simulink model "OBCSystem"  (R2025b)
settings: Solver=FixedStepAuto  StartTime=0.0  StopTime=100e-3  RelTol=1e-3  EnableMultiTasking=on
PreLoadFcn:
  | %% Load OBCSystem initialization parameters
  | initScriptPath = fullfile(fileparts(which('OBCSystem')), '..', 'SupportFiles', 'Scripts', 'OBCSystem_init.m');
  | if isfile(initScriptPath)
  |     evalin('base', fileread(initScriptPath));
  | else
  |     warning('OBCSystem:initNotFound', 'OBCSystem_init.m not found at: %s', initScriptPath);
  | end
InitFcn:
  | mode = str2double(get_param('OBCSystem/System/SimulationMode','value'));
  | enableLogging = str2double(get_param('OBCSystem/System/On-Board Charger/HIL/EnableHighResLogging','value'));
  | 
  | % If the charger runs on the FPGA AND high-resolution logging is enabled,
  | % uncomment interrupt setup. Comment otherwise
  | if ((mode == 2) && (enableLogging == 1))
  |     set_param('OBCSystem/Interrupt Setup','Commented','off');
  | else
  |     set_param('OBCSystem/Interrupt Setup','Commented','on');
  | end
  | 
  | % If DMA streaming is enambled and simulation time exceeds 30s, then throw an error
  | maxStopTime = 30;   % seconds
  | stopTimeStr = get_param(bdroot, 'StopTime');
  | stopTimeVal = str2double(stopTimeStr);
  | 
  | if enableLogging && stopTimeVal > maxStopTime
  |     error('DMA streaming is enabled, but StopTime = %.3f s exceeds the allowed %.3f s.', ...
  |           stopTimeVal, maxStopTime);
  | end
undefined symbols (not defined in the file): DAB, DAB_CCCV_Ki, DAB_CCCV_Kp, DAB_CCCV_Kt, DAB_Charging, DAB_CurrentReference, DAB_DCOffset, DAB_PhaseShift_LowerSat, DAB_PhaseShift_UpperSat, DAB_PhaseShiftInit, DAB_PhaseToDeg, DAB_PID_Kd, DAB_PID_Ki, DAB_PID_Kp, DAB_PID_LowerSat, DAB_PID_N, DAB_PID_UpperSat, Fourier_class, FPGA, FrameSize, getfullname, grid, Instr_EffGain, Instr_PinGain, Instr_PoutGain, Instr_pUtoDeg, Instr_RippleGain, Instr_SoCGain, IO334, Ki_current, Ki_voltage, Kp_current, Kp_voltage, MIL_or_HIL, OBC_template1, OpenLoopDuty, OpenLoopEnable, PCIe_RT, PFC_Current_Kb, PFC_Current_LowerSat, PFC_Current_UpperSat, PFC_Sat_DC_Lower, PFC_Sat_DC_Upper, PFC_Sat_iL_Lower, PFC_Sat_iL_Upper, PFC_Sat_Pwr_Lower, PFC_Sat_Pwr_Upper, PFC_Voltage_Kb, PFC_Voltage_LowerSat, PFC_Voltage_UpperSat, Rblock, Real, Time, totemPole, ts_CPU, ts_FPGA_clk, ts_FPGA_mdl, VectorSize
libraries: nesl_utility x27, fl_lib x24, speedgoatlib_hdlCoder_IO3xx x20, ee_lib x12, simulink x4, eeGeneralControl x4, slpidlib x3, pwm_cpulib x2, batteryecm_lib x2, slrealtimeloglib x2, pwm_fpgalib x2, speedgoatlib_interrupt x1
(part 1 of 4)
settings Model: ExtModeEnableFloating=off  ExtModeTrigDuration=100000  Creator=The MathWorks, Inc.  LastModifiedBy=aldiyar.semedyarov
settings SolverCC: ConcurrentTasks=on  AlgebraicLoopSolver=TrustRegion  PositivePriorityOrder=on  InsertRTBMode=Never (minimum delay)
settings DataIOCC: SaveFormat=Array  SaveState=on  LoggingFileName=OBCSystem_log
settings OptimizationCC: BlockReduction=off  BooleanDataType=off  GainParamInheritBuiltInType=on  OptimizeBlockIOStorage=off  BufferReuse=off  ReuseModelBlockBuffer=off  GlobalBufferReuse=off  ExpressionFolding=off  LocalBlockOutputs=off  InitFltsAndDblsToZero=on  OptimizeDataStoreBuffers=off  BusAssignmentInplaceUpdate=off
settings DebuggingCC: SaveWithParameterizedLinksMsg=none  UnderspecifiedInitializationDetection=Classic  MergeDetectMultiDrivingBlocksExec=none  CheckExecutionContextPreStartOutputMsg=on  SignalResolutionControl=TryResolveAllWithWarning  InheritedTsInSrcMsg=none  TasksWithSamePriorityMsg=none  UnconnectedInputMsg=warning  UnconnectedOutputMsg=warning  UnconnectedLineMsg=warning  SFUnexpectedBacktrackingDiag=warning  SFNoUnconditionalDefaultTransitionDiag=warning  SFExecutionAtInitializationDiag=none  ArithmeticOperatorsInVariantConditions=warning
settings HardwareCC: ProdBitPerLong=64.0  ProdLongLongMode=on  ProdHWDeviceType=Intel->x86-64 (Linux 64)
settings ModelReferenceCC: EnableRefExpFcnMdlSchedulingChecks=on  PropagateSignalLabelsOutOfModel=off
settings SFSimCC: SimUseLocalCustomCode=off  CustomCodeUndefinedFunction=UseInterfaceOnly
settings RTWCC: SystemTargetFile=speedgoat.tlc  TemplateMakefile=slrealtime_default_tmf  RTWUseLocalCustomCode=off  Toolchain=Simulink Real-Time Toolchain  BuildConfiguration=Faster Runs  CodeExecutionProfiling=on  TargetLang=C++  GPUComputeCapability=3.5  Description=Speedgoat Real-Time Target Machine
settings CodeAppCC: StateflowObjectComments=on
settings SimulinkRealTimeTargetCC: SLRTFileLogMaxRuns=1.0  ExtModeMaxTrigDuration=10.0  ExtModeStaticAllocSize=1000000.0  ExtModeTransport=0.0  MultiwordLength=2048.0  DynamicStringBufferSize=256.0  PreserveMATLABNamespacesInGeneratedCode=on  SubcomponentCodeInterfacePackaging=Reusable function  MATLABClassNameForMDSCustomization=Simulink.SoftwareTarget.GRTCustomization  InstructionSetFMA=off  LogToMDFFile=off
settings ConfigComp: CovMetricSettings=dw  CovSaveCumulativeToWorkspaceVar=on  CovSaveSingleToWorkspaceVar=on  CovExternalEMLEnable=off  CovSFcnEnable=off

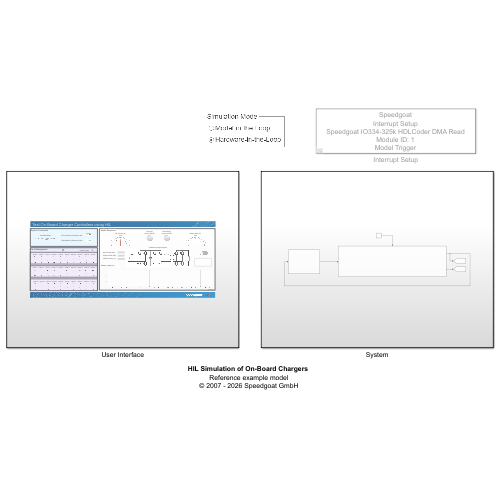
[thumbnail: Simulink's stored preview of the top-level diagram]
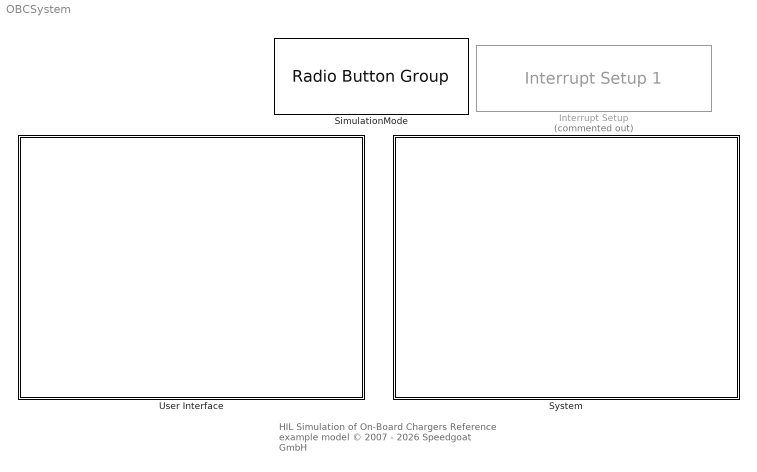
== system OBCSystem ==
  note: HIL Simulation of On-Board Chargers
      | Reference example model
      | © 2007 - 2026 Speedgoat GmbH
  Interrupt Setup : speedgoatlib_interrupt/Interrupt Setup 1  Commented=on  parModuleTrigger=on  parPollingMode=off  parPriorityConf=High  parPriority=253  confStartFcn=IO334_325K_HDLC_DMA_READ_start_public  confStopFcn=IO334_325K_HDLC_DMA_READ_stop_public  confIsrFcn=IO334_325K_HDLC_DMA_READ_isr_public  confMapFcn=IO334_325K_HDLC_DMA_READ_map_public  confHookFile=io334_325k_hdlc_dma_read_int_hooks.c  confIrqNr=-1  confIsPolling=off  confModID=16776961  confSelectedInt=Speedgoat IO334-325k HDLCoder DMA Read  confSelectedId=1  confSelectedChannel=[]  confData=[90 1]  confForcePollingMode=off
  SimulationMode : RadioButtonGroup  LabelPosition=Hide  SelectedLabel=Hardware-in-the-Loop  ButtonGroupName=Simulation Mode
  System : Subsystem
  User Interface : Subsystem

== system OBCSystem/System ==
  Controller : Subsystem
  On-Board Charger : Subsystem  Variant=on  VariantControl=Choice
      settings: PortSchema="{\"entries\":[{\"content\":{\"sides\":[{\"content\":{\"connectorIds\":[\"In1\"]},\"type\":\"ConnectorPlacement.EquallySpacedRectSide\",\"uuid\":\"470e74a6-3489-4910-833e-9935ca68db72\"},{\"content\":{\"connectorIds\":[\"Out1\",\"Out2\"],\"side\":\"RIGHT\"},\"type\":\"ConnectorPlacement.EquallySpacedRectSide\",\"uuid\":\"2bffa5e5-f1a3-4939-a790-ed9d5415056f\"},{\"content\":{\"connectorIds\":[\"In2\"],\"side\":\"TOP\"},\"type\":\"ConnectorPlacement.EquallySpacedRectSide\",\"uuid\":\"16820d5e-786f-42c5-b0ca-13ece32c30be\"}]},\"type\":\"ConnectorPlacement.EquallySpacedConnector\",\"uuid\":\"b4a77eb5-3b93-4396-97dc-6ff44775ea65\"}],\"packageUris\":[\"http://schema.mathworks.com/mf0/Connector/R2020b\"],\"version\":\"1.0\"}"
      mask Display: image('OnboardChargerSchematics.png');
  SimulationMode : Constant  Value=2  OutDataTypeStr=single  SampleTime=ts_CPU
  tag scope: Meas_bus2=global, Meas_bus=global
  wires:
  Controller/1(PWM_bus) -> On-Board Charger/1(PWM_bus)
  SimulationMode/1 -> On-Board Charger/2(Mode)
  On-Board Charger/1(Meas_bus) -> [Meas_bus], Controller/1(Meas_bus)
  On-Board Charger/2(Meas_bus2) -> [Meas_bus2]

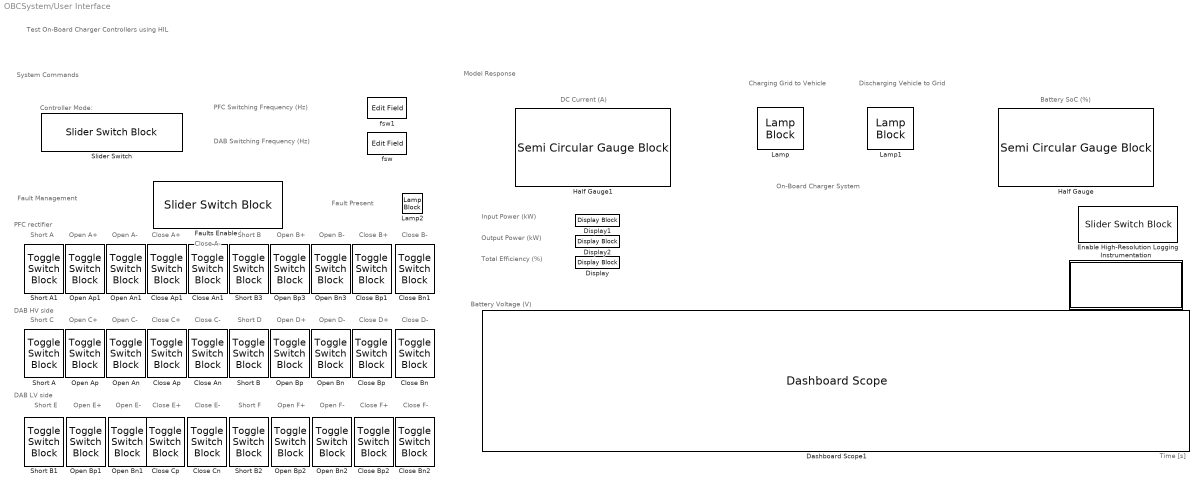
== system OBCSystem/User Interface ==
  note: Open C-
  note: PFC rectifier
  note: Open E-
  note: System Commands
  note: Short E
  note: Close D+
  note: Short F
  note: Discharging
      | Vehicle to Grid
  note: Model Response
  note: Close E-
  note: DC Current (A)
  note: Fault Present
  note: Charging
      | Grid to Vehicle
  note: Controller Mode:
  note: DAB HV side
  note: Open F-
  note: Battery Voltage (V)
  note: Open D-
  note: On-Board Charger System
  note: Open E+
  note: Close C+
  note: Close D-
  note: Fault Management
  note: DAB Switching Frequency (Hz)
  note: Short C
  note: Short D
  note: Close A-
  note: Battery SoC (%)
  note: Open B+
  note: Short A
  note: Close A+
  note: Close B+
  note: Short B
  note: Time [s]
  note: Close F-
  note: DAB LV side
  note: Open F+
  note: Open D+
  note: Close C-
  note: Open B-
  note: Close B-
  note: Close E+
  note: Open A+
  note: Open A-
  note: Close F+
  note: Test On-Board Charger Controllers using HIL
  note: PFC Switching Frequency (Hz)
  note: Open C+
  note: Total Efficiency (%)
  note: Input Power (kW)
  note: Output Power (kW)
  Close An : ToggleSwitchBlock  LabelPosition=Hide
  Close An1 : ToggleSwitchBlock  LabelPosition=Hide
  Close Ap : ToggleSwitchBlock  LabelPosition=Hide
  Close Ap1 : ToggleSwitchBlock  LabelPosition=Hide
  Close Bn : ToggleSwitchBlock  LabelPosition=Hide
  Close Bn1 : ToggleSwitchBlock  LabelPosition=Hide
  Close Bn2 : ToggleSwitchBlock  LabelPosition=Hide
  Close Bp : ToggleSwitchBlock  LabelPosition=Hide
  Close Bp1 : ToggleSwitchBlock  LabelPosition=Hide
  Close Bp2 : ToggleSwitchBlock  LabelPosition=Hide
  Close Cn : ToggleSwitchBlock  LabelPosition=Hide
  Close Cp : ToggleSwitchBlock  LabelPosition=Hide
  Dashboard Scope1 : DashboardScope  ShowInitialText=off  TimeSpan=45  Ymin=385  Ymax=402.5  ScaleAtStop=off  FontColor=[0.0, 0.0, 0.0]
  Display : DisplayBlock  LabelPosition=Hide  Transparency=1  GridColor=[0.502, 0.502, 0.502]
  Display1 : DisplayBlock  LabelPosition=Hide  Transparency=1  GridColor=[0.502, 0.502, 0.502]
  Display2 : DisplayBlock  LabelPosition=Hide  Transparency=1  GridColor=[0.502, 0.502, 0.502]
  Enable High-Resolution Logging : SliderSwitchBlock  LabelPosition=Hide
  Faults Enabled : SliderSwitchBlock  LabelPosition=Hide
  Half Gauge : SemiCircularGaugeBlock  LabelPosition=Hide  FontColor=[0.0, 0.0, 0.0]
  Half Gauge1 : SemiCircularGaugeBlock  LabelPosition=Hide  ScaleMin=-20  ScaleMax=20  FontColor=[0.0, 0.0, 0.0]
  Instrumentation : Subsystem
  Lamp : LampBlock  LabelPosition=Hide  DefaultColor=[192.0, 192.0, 192.0]
  Lamp1 : LampBlock  LabelPosition=Hide  DefaultColor=[192.0, 192.0, 192.0]
  Lamp2 : LampBlock  LabelPosition=Hide  DefaultColor=[192.0, 192.0, 192.0]
  Open An : ToggleSwitchBlock  LabelPosition=Hide
  Open An1 : ToggleSwitchBlock  LabelPosition=Hide
  Open Ap : ToggleSwitchBlock  LabelPosition=Hide
  Open Ap1 : ToggleSwitchBlock  LabelPosition=Hide
  Open Bn{,1..3} (4 alike) : ToggleSwitchBlock  LabelPosition=Hide
  Open Bp{,1..3} (4 alike) : ToggleSwitchBlock  LabelPosition=Hide
  Short A : ToggleSwitchBlock  LabelPosition=Hide
  Short A1 : ToggleSwitchBlock  LabelPosition=Hide
  Short B{,1..3} (4 alike) : ToggleSwitchBlock  LabelPosition=Hide
  Slider Switch : SliderSwitchBlock  LabelPosition=Hide
  fsw : EditField  LabelPosition=Hide  ShowInitialText=on  Alignment=Center
  fsw1 : EditField  LabelPosition=Hide  ShowInitialText=on  Alignment=Center

== system OBCSystem/System/Controller ==
  Meas_bus : Inport
  Bus Creator : BusCreator  Inputs=4
  Bus Selector : BusSelector  OutputSignals=VCbus,iL_PFC,Vs,Ibatt,Vbatt
  DAB Controller : Subsystem
  Ibatt_ref : Constant  Value=DAB_CurrentReference  OutDataTypeStr=double  SampleTime=ts_CPU
  PFC Controller : Subsystem
  PFC Reference DC Voltage : Constant  Value=400  OutDataTypeStr=single  SampleTime=ts_CPU
  PWM_bus : Outport
  tag scope: Ibatt_ref=global, Vdc_ref=global
  wires:
  Bus Selector/2 -> PFC Controller/3(Measured inductor current)  "<iL_PFC>"
  PFC Reference DC Voltage/1 -> [Vdc_ref]
  Bus Selector/3 -> PFC Controller/4(Source voltage)  "<Vs>"
  Bus Selector/5 -> DAB Controller/2(Measured battery voltage)  "<Vbatt>"
  Meas_bus/1 -> Bus Selector/1
  Bus Selector/1 -> PFC Controller/2(Measured bus voltage)  "<VCbus>"
  [Vdc_ref] -> PFC Controller/1(Reference bus voltage)
  PFC Controller/1(PWM_Config_PFC) -> Bus Creator/1  "PWM_Config_PFC"
  PFC Controller/2(PWM_Runtime_PFC) -> Bus Creator/2  "PWM_Runtime_PFC"
  DAB Controller/1(PWM_Config_DAB) -> Bus Creator/3  "PWM_Config_DAB"
  DAB Controller/2(PWM_Runtime_DAB) -> Bus Creator/4  "PWM_Runtime_DAB"
  Bus Creator/1 -> PWM_bus/1
  Ibatt_ref/1 -> [Ibatt_ref]
  [Ibatt_ref] -> DAB Controller/3(Reference battery current)
  Bus Selector/4 -> DAB Controller/1(Measured battery current)  "<Ibatt>"

== system OBCSystem/System/On-Board Charger ==
  PWM_bus : Inport
  Mode : Inport  Port=2
  HIL : Subsystem  VariantControl=strcmp(get_param('OBCSystem/System/SimulationMode','value'),'2')
  MIL : Subsystem  VariantControl=strcmp(get_param('OBCSystem/System/SimulationMode','value'),'1')
  Meas_bus : Outport
  Meas_bus2 : Outport  Port=2

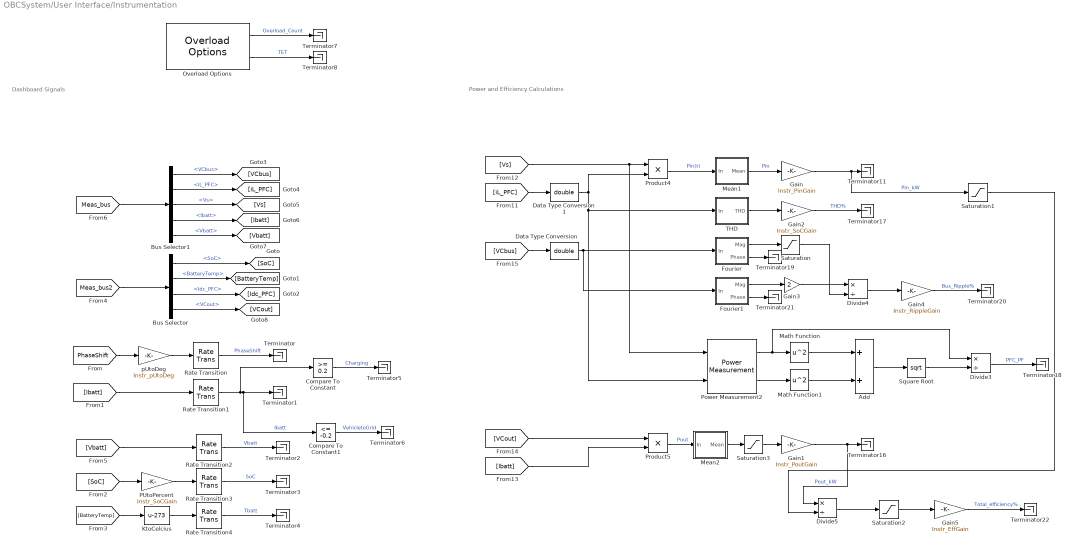
== system OBCSystem/User Interface/Instrumentation ==
  note: Dashboard Signals
  note: Power and Efficiency Calculations
  Add : Sum
  Bus Selector : BusSelector  OutputSignals=SoC,BatteryTemp,Idc_PFC,VCout
  Bus Selector1 : BusSelector  OutputSignals=VCbus,iL_PFC,Vs,Ibatt,Vbatt
  Compare To Constant : simulink/Logic and Bit Operations/Compare To Constant  relop=>=  const=0.2  OutDataTypeStr=boolean
  Compare To Constant1 : simulink/Logic and Bit Operations/Compare To Constant  relop=<=  const=-0.2  OutDataTypeStr=boolean
  Data Type Conversion : DataTypeConversion  OutDataTypeStr=double  SaturateOnIntegerOverflow=off  RndMeth=Floor
  Data Type Conversion1 : DataTypeConversion  OutDataTypeStr=double  SaturateOnIntegerOverflow=off  RndMeth=Floor
  Divide3 : Product  Inputs=*/
  Divide4 : Product  Inputs=*/
  Divide5 : Product  Inputs=*/
  Fourier : Subsystem
      settings: OpenFcn=elec.conv.unmask(gcb);
  Fourier1 : Subsystem
  Gain : Gain  Gain=Instr_PinGain
  Gain1 : Gain  Gain=Instr_PoutGain
  Gain2 : Gain  Gain=Instr_SoCGain
  Gain3 : Gain  Gain=2
  Gain4 : Gain  Gain=Instr_RippleGain
  Gain5 : Gain  Gain=Instr_EffGain
  KtoCelcius : Bias  Bias=-273  SaturateOnIntegerOverflow=off
  Math Function : Math  Operator=square
  Math Function1 : Math  Operator=square
  Mean1 : Subsystem
  Mean2 : Subsystem
      settings: OpenFcn=elec.conv.unmask(gcb);
  Overload Options : slrealtimetgmanagement/Overload Options  startupDur=1  startupDurSrc=Tunable Parameter  maxOverload=100  maxOverloadSrc=Tunable Parameter  TETFlag=on
  PUtoPercent : Gain  Gain=Instr_SoCGain
  Power Measurement2 : eePowerMeasurement/Power Measurement  LabelModeActiveChoice=Discrete  F=50  K=1  Ts=ts_CPU
  Product4 : Product  OutDataTypeStr=double
  Product5 : Product  OutDataTypeStr=double
  Rate Transition : RateTransition  OutPortSampleTime=1e-3
  Rate Transition1 : RateTransition  OutPortSampleTime=1e-3
  Rate Transition2 : RateTransition  InitialCondition=386  OutPortSampleTime=1e-3
  Rate Transition3 : RateTransition  InitialCondition=0.75  OutPortSampleTime=1e-3
  Rate Transition4 : RateTransition  InitialCondition=20  OutPortSampleTime=1e-3
  Saturation : Saturate  UpperLimit=inf  LowerLimit=eps
  Saturation1 : Saturate  UpperLimit=inf  LowerLimit=eps
  Saturation2 : Saturate  UpperLimit=1  LowerLimit=0
  Saturation3 : Saturate  UpperLimit=inf  LowerLimit=0
  Square Root : Sqrt
  THD : Subsystem
  Terminator{,1..8,11,16..22} (17 alike) : Terminator
  pUtoDeg : Gain  Gain=Instr_pUtoDeg
  wires:
  [PhaseShift] -> pUtoDeg/1
  [Ibatt] -> Rate Transition1/1
  [Vbatt] -> Rate Transition2/1
  Rate Transition/1 -> Terminator/1  "PhaseShift"
  Rate Transition1/1 -> Compare To Constant/1, Compare To Constant1/1, Terminator1/1  "Ibatt"
  Rate Transition2/1 -> Terminator2/1  "Vbatt"
  Rate Transition3/1 -> Terminator3/1  "SoC"
  pUtoDeg/1 -> Rate Transition/1
  [SoC] -> PUtoPercent/1
  [BatteryTemp] -> KtoCelcius/1
  Rate Transition4/1 -> Terminator4/1  "Tbatt"
  KtoCelcius/1 -> Rate Transition4/1
  Compare To Constant/1 -> Terminator5/1  "Charging"
  Compare To Constant1/1 -> Terminator6/1  "VehicletoGrid"
  PUtoPercent/1 -> Rate Transition3/1
  Overload Options/1 -> Terminator7/1  "Overload_Count"
  Overload Options/2 -> Terminator8/1  "TET"
  [Vs] -> Power Measurement2/1, Product4/1
  [iL_PFC] -> Data Type Conversion1/1
  Mean1/1(Mean) -> Gain/1  "Pin"
  Product4/1 -> Mean1/1(In)  "Pin(t)"
  Gain/1 -> Saturation1/1, Terminator11/1  "Pin_kW"
  Gain1/1 -> Divide5/1, Terminator16/1  "Pout_kW"
  [Ibatt] -> Product5/2
  [VCout] -> Product5/1
  THD/1(THD) -> Gain2/1
  Gain2/1 -> Terminator17/1  "THD%"
  Power Measurement2/1 -> Divide3/1, Math Function/1
  Math Function/1 -> Add/1
  Power Measurement2/2 -> Math Function1/1
  Math Function1/1 -> Add/2
  Add/1 -> Square Root/1
  Square Root/1 -> Divide3/2
  Divide3/1 -> Terminator18/1  "PFC_PF"
  [VCbus] -> Data Type Conversion/1
  Fourier/1(Mag) -> Saturation/1
  Fourier/2(Phase) -> Terminator19/1
  Gain3/1 -> Divide4/1
  Saturation/1 -> Divide4/2
  Fourier1/1(Mag) -> Gain3/1
  Divide4/1 -> Gain4/1
  Gain4/1 -> Terminator20/1  "Bus_Ripple%"
  Fourier1/2(Phase) -> Terminator21/1
  Data Type Conversion/1 -> Fourier1/1(In), Fourier/1(In)
  Data Type Conversion1/1 -> Power Measurement2/2, THD/1(In), Product4/2
  Divide5/1 -> Saturation2/1
  Gain5/1 -> Terminator22/1  "Total_efficiency%"
  Saturation2/1 -> Gain5/1
  Saturation1/1 -> Divide5/2
  [Meas_bus2] -> Bus Selector/1
  Bus Selector/1 -> [SoC]  "<SoC>"
  Bus Selector/2 -> [BatteryTemp]  "<BatteryTemp>"
  Bus Selector/3 -> [Idc_PFC]  "<Idc_PFC>"
  [Meas_bus] -> Bus Selector1/1
  Bus Selector1/1 -> [VCbus]  "<VCbus>"
  Bus Selector1/2 -> [iL_PFC]  "<iL_PFC>"
  Bus Selector1/3 -> [Vs]  "<Vs>"
  Bus Selector1/4 -> [Ibatt]  "<Ibatt>"
  Bus Selector1/5 -> [Vbatt]  "<Vbatt>"
  Bus Selector/4 -> [VCout]  "<VCout>"
  Product5/1 -> Mean2/1(In)  "Pout"
  Mean2/1(Mean) -> Saturation3/1
  Saturation3/1 -> Gain1/1

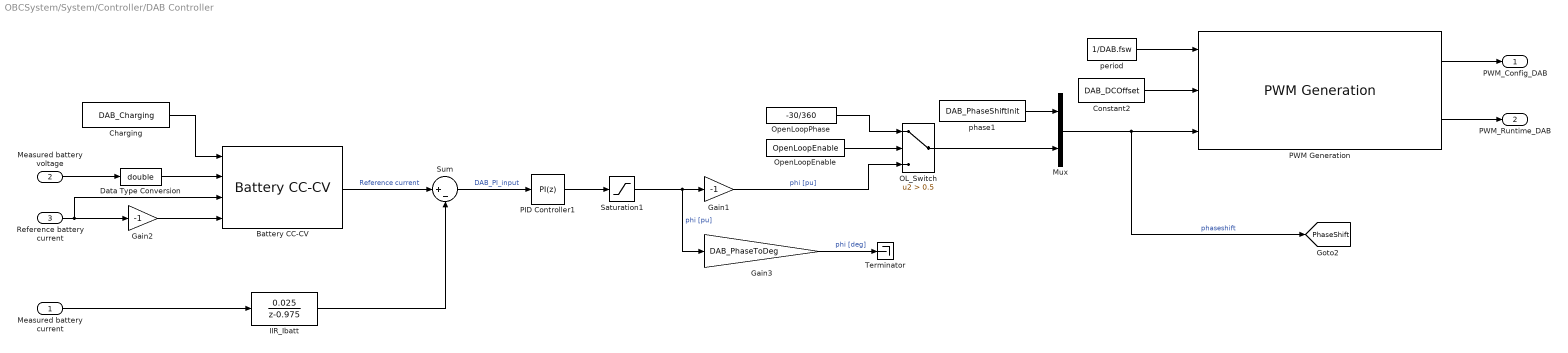
== system OBCSystem/System/Controller/DAB Controller ==
  Measured battery current : Inport
  Measured battery voltage : Inport  Port=2
  Reference battery current : Inport  Port=3
  Battery CC-CV : BatteryCurrentManagement/Battery CC-CV  MinMaxFlag=off  MaxCellVoltage=MaxCellVoltage  Kp=DAB_CCCV_Kp  Ki=DAB_CCCV_Ki  Kaw=DAB_CCCV_Kaw  Kt=DAB_CCCV_Kt  Ts=-1
      settings: LibrarySourceBlock=batt_sl_lib/Current Management/Battery CC-CV
  Charging : Constant  Value=DAB_Charging  SampleTime=ts_CPU
  Constant2 : Constant  Value=DAB_DCOffset  SampleTime=-1
  Data Type Conversion : DataTypeConversion  OutDataTypeStr=double  SaturateOnIntegerOverflow=off  RndMeth=Floor
  Gain1 : Gain  Gain=-1
  Gain2 : Gain  Gain=-1
  Gain3 : Gain  Gain=DAB_PhaseToDeg
  IIR_Ibatt : DiscreteTransferFcn  Numerator=[0.025]  Denominator=[1, -0.975]  SampleTime=ts_CPU
  Mux : Mux  Inputs=2
  OL_Switch : Switch  Criteria=u2 > Threshold  Threshold=0.5  SaturateOnIntegerOverflow=off  InputSameDT=off
  OpenLoopEnable : Constant  Value=OpenLoopEnable  SampleTime=ts_CPU
  OpenLoopPhase : Constant  Value=-30/360  SampleTime=ts_CPU
  PID Controller1 : slpidlib/PID Controller  Controller=PI  Form=Parallel  TimeDomain=Discrete-time  UseExternalTs=off  SampleTime=ts_CPU  IntegratorMethod=Forward Euler  FilterMethod=Forward Euler  ControllerParametersSource=internal  P=DAB_PID_Kp  I=DAB_PID_Ki  UseKiTs=off  D=DAB_PID_Kd  UseExternalDerivativeSource=off  N=DAB_PID_N  UseFilter=on  TunerSelectOption=Transfer Function Based (PID Tuner App)  InitialConditionSource=internal  InitialConditionForIntegrator=0  InitialConditionForFilter=0  DifferentiatorICPrevScaledInput=0  ExternalReset=none  TrackingMode=off  Kt=1  LimitOutput=on  SatLimitsSource=internal  UpperSaturationLimit=DAB_PID_UpperSat  LowerSaturationLimit=DAB_PID_LowerSat  LinearizeAsGain=on  AntiWindupMode=clamping  Kb=1  LimitIntegrator=off  UpperIntegratorSaturationLimit=inf  LowerIntegratorSaturationLimit=-inf  POutMin=[]  POutMax=[]  IOutMin=[]  IOutMax=[]  DOutMin=[]  DOutMax=[]  NOutMin=[]  NOutMax=[]  SumOutMin=[]  SumOutMax=[]  SaturationOutMin=[]  SaturationOutMax=[]  PParamMin=[]  PParamMax=[]  IParamMin=[]  IParamMax=[]  DParamMin=[]  DParamMax=[]  NParamMin=[]  NParamMax=[]  KbParamMin=[]  KbParamMax=[]  KtParamMin=[]  KtParamMax=[]  KbOutMin=[]  KbOutMax=[]  KtOutMin=[]  KtOutMax=[]  IntegratorOutMin=[]  IntegratorOutMax=[]  FilterOutMin=[]  FilterOutMax=[]  SumI1OutMin=[]  SumI1OutMax=[]  SumI2OutMin=[]  SumI2OutMax=[]  SumI3OutMin=[]  SumI3OutMax=[]  SumI4OutMin=[]  SumI4OutMax=[]  SumDOutMin=[]  SumDOutMax=[]  DifferentiatorOutMin=[]  DifferentiatorOutMax=[]  FilterDiffOutCoefMin=[]  FilterDiffOutCoefMax=[]  ReciprocalOutMin=[]  ReciprocalOutMax=[]  SumDenOutMin=[]  SumDenOutMax=[]  SumNumOutMin=[]  SumNumOutMax=[]  DivideOutMin=[]  DivideOutMax=[]  UdiffTsProdOutMin=[]  UdiffTsProdOutMax=[]  NTsProdOutMin=[]  NTsProdOutMax=[]  UintegralTsProdOutMin=[]  UintegralTsProdOutMax=[]  UngainTsProdOutMin=[]  UngainTsProdOutMax=[]  ClampingZeroOutDataTypeStr=Inherit: Inherit via back propagation  ClampingZeroOutMin=[]  ClampingZeroOutMax=[]  FilterDenConstantOutDataTypeStr=Inherit: Inherit via back propagation  FilterDenConstantOutMin=[]  FilterDenConstantOutMax=[]  PCopyOutDataTypeStr=Inherit: Inherit via back propagation  PCopyOutMin=[]  PCopyOutMax=[]  NCopyOutDataTypeStr=Inherit: Inherit via back propagation  NCopyOutMin=[]  NCopyOutMax=[]  IntegratorContinuousStateAttributes=''  IntegratorStateMustResolveToSignalObject=off  IntegratorRTWStateStorageClass=Auto  FilterContinuousStateAttributes=''  FilterStateMustResolveToSignalObject=off  FilterRTWStateStorageClass=Auto  ParallelPVariant=InternalParameters  IdealPVariant=Disabled  IVariant=InternalParameters  DVariant=Disabled  IntegratorVariant=Discrete  SatVariant=Enabled  AWVariant=DiscClampingParallel  PCopyVariant=Disabled  TRVariant=Disabled  FdbkBlocksVariant=Forward  IdealPFdbkVariant=Disabled  SatFdbkVariant=Disabled  DerivativeFilterVariant=Disabled  NVariant=Disabled  NCopyVariant=Disabled_SignalSpec  FilterICVariant=Disabled  IntegratorICVariant=InternalICs  ExternalResetVariant=Disabled  TRSumVariant=Passthrough  SumFdbkVariant=Disabled  SumVariant=Sum_PI  TsampFilterVariant=InternalTs  TsampNgainVariant=Passthrough  TsampIntegralVariant=Disabled_SignalSpec  ExternalSaturationOutDataTypeStr=Inherit: Same as second input  DerivativeSourceVariant=Disabled  PreIntVariant=InternalPreInt
  PWM Generation : pwm_cpulib/PWM Generation  f_FPGA=1/ts_FPGA_clk  n_channels=2  sel_scaling=CPU  protection_param=B is forced off when A is on.  deadband_sec=DAB_PWM_Deadband  natural_update=At period starts  delay=0  trigger_duration_sec=[1e-6]  trigger_period_start=off  trigger_half_of_the_period=off  trigger_a_on=off  trigger_a_off=off  trigger_b_on=off  trigger_b_off=off  bit_width_pwm_gen=DAB_PWM_BitWidth  invert_a=off  invert_b=off  invert_c=off  showPhaseInput=on
      settings: SourceProductName=PWM CPU Library
  Saturation1 : Saturate  UpperLimit=DAB_PhaseShift_UpperSat  LowerLimit=DAB_PhaseShift_LowerSat
  Sum : Sum  Inputs=|+-
  Terminator : Terminator
  period : Constant  Value=1/DAB.fsw  SampleTime=-1
  phase1 : Constant  Value=DAB_PhaseShiftInit  SampleTime=-1
  PWM_Config_DAB : Outport  VectorParamsAs1DForOutWhenUnconnected=off
  PWM_Runtime_DAB : Outport  Port=2  VectorParamsAs1DForOutWhenUnconnected=off
  tag scope: PhaseShift=global
  wires:
  Sum/1 -> PID Controller1/1  "DAB_PI_input"
  Saturation1/1 -> Gain1/1, Gain3/1  "phi [pu]"
  PID Controller1/1 -> Saturation1/1
  Measured battery current/1 -> IIR_Ibatt/1
  Gain3/1 -> Terminator/1  "phi [deg]"
  period/1 -> PWM Generation/1
  phase1/1 -> Mux/1
  Mux/1 -> PWM Generation/3, [PhaseShift]  "phaseshift"
  Constant2/1 -> PWM Generation/2
  PWM Generation/1 -> PWM_Config_DAB/1
  PWM Generation/2 -> PWM_Runtime_DAB/1
  Gain1/1 -> OL_Switch/3  "phi [pu]"
  Measured battery voltage/1 -> Data Type Conversion/1
  Gain2/1 -> Battery CC-CV/4
  Battery CC-CV/1 -> Sum/1  "Reference current"
  Charging/1 -> Battery CC-CV/1
  IIR_Ibatt/1 -> Sum/2
  Reference battery current/1 -> Gain2/1, Battery CC-CV/3
  Data Type Conversion/1 -> Battery CC-CV/2
  OpenLoopPhase/1 -> OL_Switch/1
  OL_Switch/1 -> Mux/2
  OpenLoopEnable/1 -> OL_Switch/2

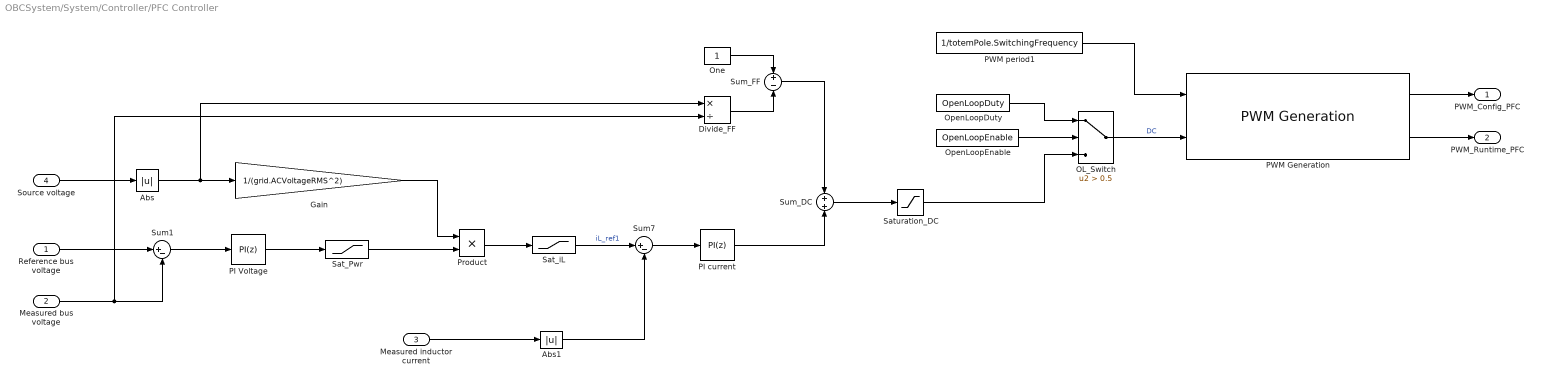
== system OBCSystem/System/Controller/PFC Controller ==
  Reference bus voltage : Inport
  Measured bus voltage : Inport  Port=2
  Measured inductor current : Inport  Port=3
  Source voltage : Inport  Port=4
  Abs : Abs  SaturateOnIntegerOverflow=off
  Abs1 : Abs  SaturateOnIntegerOverflow=off
  Divide_FF : Product  Inputs=*/
  Gain : Gain  Gain=1/(grid.ACVoltageRMS^2)
  OL_Switch : Switch  Criteria=u2 > Threshold  Threshold=0.5  SaturateOnIntegerOverflow=off  InputSameDT=off
  One : Constant  SampleTime=ts_CPU
  OpenLoopDuty : Constant  Value=OpenLoopDuty  SampleTime=ts_CPU
  OpenLoopEnable : Constant  Value=OpenLoopEnable  SampleTime=ts_CPU
  PI Voltage : slpidlib/PID Controller  Controller=PI  Form=Parallel  TimeDomain=Discrete-time  UseExternalTs=off  SampleTime=ts_CPU  IntegratorMethod=Backward Euler  FilterMethod=Forward Euler  ControllerParametersSource=internal  P=Kp_voltage  I=Ki_voltage  UseKiTs=off  D=8.78727522810553e-08  UseExternalDerivativeSource=off  N=100  UseFilter=on  TunerSelectOption=Transfer Function Based (PID Tuner App)  InitialConditionSource=internal  InitialConditionForIntegrator=0  InitialConditionForFilter=0  DifferentiatorICPrevScaledInput=0  ExternalReset=none  TrackingMode=off  Kt=1  LimitOutput=on  SatLimitsSource=internal  UpperSaturationLimit=PFC_Voltage_UpperSat  LowerSaturationLimit=PFC_Voltage_LowerSat  LinearizeAsGain=off  AntiWindupMode=back-calculation  Kb=PFC_Voltage_Kb  LimitIntegrator=on  UpperIntegratorSaturationLimit=7500  LowerIntegratorSaturationLimit=-1000  POutMin=[]  POutMax=[]  IOutMin=[]  IOutMax=[]  DOutMin=[]  DOutMax=[]  NOutMin=[]  NOutMax=[]  SumOutMin=[]  SumOutMax=[]  SaturationOutMin=[]  SaturationOutMax=[]  PParamMin=[]  PParamMax=[]  IParamMin=[]  IParamMax=[]  DParamMin=[]  DParamMax=[]  NParamMin=[]  NParamMax=[]  KbParamMin=[]  KbParamMax=[]  KtParamMin=[]  KtParamMax=[]  KbOutMin=[]  KbOutMax=[]  KtOutMin=[]  KtOutMax=[]  IntegratorOutMin=[]  IntegratorOutMax=[]  FilterOutMin=[]  FilterOutMax=[]  SumI1OutMin=[]  SumI1OutMax=[]  SumI2OutMin=[]  SumI2OutMax=[]  SumI3OutMin=[]  SumI3OutMax=[]  SumI4OutMin=[]  SumI4OutMax=[]  SumDOutMin=[]  SumDOutMax=[]  DifferentiatorOutMin=[]  DifferentiatorOutMax=[]  FilterDiffOutCoefMin=[]  FilterDiffOutCoefMax=[]  ReciprocalOutMin=[]  ReciprocalOutMax=[]  SumDenOutMin=[]  SumDenOutMax=[]  SumNumOutMin=[]  SumNumOutMax=[]  DivideOutMin=[]  DivideOutMax=[]  UdiffTsProdOutMin=[]  UdiffTsProdOutMax=[]  NTsProdOutMin=[]  NTsProdOutMax=[]  UintegralTsProdOutMin=[]  UintegralTsProdOutMax=[]  UngainTsProdOutMin=[]  UngainTsProdOutMax=[]  ClampingZeroOutDataTypeStr=Inherit: Inherit via back propagation  ClampingZeroOutMin=[]  ClampingZeroOutMax=[]  FilterDenConstantOutDataTypeStr=Inherit: Inherit via back propagation  FilterDenConstantOutMin=[]  FilterDenConstantOutMax=[]  PCopyOutDataTypeStr=Inherit: Inherit via back propagation  PCopyOutMin=[]  PCopyOutMax=[]  NCopyOutDataTypeStr=Inherit: Inherit via back propagation  NCopyOutMin=[]  NCopyOutMax=[]  IntegratorContinuousStateAttributes=''  IntegratorStateMustResolveToSignalObject=off  IntegratorRTWStateStorageClass=Auto  FilterContinuousStateAttributes=''  FilterStateMustResolveToSignalObject=off  FilterRTWStateStorageClass=Auto  ParallelPVariant=InternalParameters  IdealPVariant=Disabled  IVariant=InternalParameters  DVariant=Disabled  IntegratorVariant=Discrete  SatVariant=Enabled  AWVariant=BackCalculation  PCopyVariant=Disabled  TRVariant=Disabled  FdbkBlocksVariant=Feedback  IdealPFdbkVariant=Passthrough  SatFdbkVariant=Enabled  DerivativeFilterVariant=Disabled  NVariant=Disabled  NCopyVariant=Disabled_SignalSpec  FilterICVariant=Disabled  IntegratorICVariant=InternalICs  ExternalResetVariant=Disabled  TRSumVariant=Passthrough  SumFdbkVariant=Enabled  SumVariant=Sum_PI  TsampFilterVariant=InternalTs  TsampNgainVariant=Passthrough  TsampIntegralVariant=Disabled_SignalSpec  ExternalSaturationOutDataTypeStr=Inherit: Same as second input  DerivativeSourceVariant=Disabled  PreIntVariant=InternalPreInt
  PI current : slpidlib/PID Controller  Controller=PI  Form=Parallel  TimeDomain=Discrete-time  UseExternalTs=off  SampleTime=ts_CPU  IntegratorMethod=Backward Euler  FilterMethod=Forward Euler  ControllerParametersSource=internal  P=Kp_current  I=Ki_current  UseKiTs=off  D=0  UseExternalDerivativeSource=off  N=100  UseFilter=on  TunerSelectOption=Frequency Response Based  InitialConditionSource=internal  InitialConditionForIntegrator=0  InitialConditionForFilter=0  DifferentiatorICPrevScaledInput=0  ExternalReset=none  TrackingMode=off  Kt=1  LimitOutput=on  SatLimitsSource=internal  UpperSaturationLimit=PFC_Current_UpperSat  LowerSaturationLimit=PFC_Current_LowerSat  LinearizeAsGain=on  AntiWindupMode=back-calculation  Kb=PFC_Current_Kb  LimitIntegrator=on  UpperIntegratorSaturationLimit=1  LowerIntegratorSaturationLimit=-1  POutMin=[]  POutMax=[]  IOutMin=[]  IOutMax=[]  DOutMin=[]  DOutMax=[]  NOutMin=[]  NOutMax=[]  SumOutMin=[]  SumOutMax=[]  SaturationOutMin=[]  SaturationOutMax=[]  PParamMin=[]  PParamMax=[]  IParamMin=[]  IParamMax=[]  DParamMin=[]  DParamMax=[]  NParamMin=[]  NParamMax=[]  KbParamMin=[]  KbParamMax=[]  KtParamMin=[]  KtParamMax=[]  KbOutMin=[]  KbOutMax=[]  KtOutMin=[]  KtOutMax=[]  IntegratorOutMin=[]  IntegratorOutMax=[]  FilterOutMin=[]  FilterOutMax=[]  SumI1OutMin=[]  SumI1OutMax=[]  SumI2OutMin=[]  SumI2OutMax=[]  SumI3OutMin=[]  SumI3OutMax=[]  SumI4OutMin=[]  SumI4OutMax=[]  SumDOutMin=[]  SumDOutMax=[]  DifferentiatorOutMin=[]  DifferentiatorOutMax=[]  FilterDiffOutCoefMin=[]  FilterDiffOutCoefMax=[]  ReciprocalOutMin=[]  ReciprocalOutMax=[]  SumDenOutMin=[]  SumDenOutMax=[]  SumNumOutMin=[]  SumNumOutMax=[]  DivideOutMin=[]  DivideOutMax=[]  UdiffTsProdOutMin=[]  UdiffTsProdOutMax=[]  NTsProdOutMin=[]  NTsProdOutMax=[]  UintegralTsProdOutMin=[]  UintegralTsProdOutMax=[]  UngainTsProdOutMin=[]  UngainTsProdOutMax=[]  ClampingZeroOutDataTypeStr=Inherit: Inherit via back propagation  ClampingZeroOutMin=[]  ClampingZeroOutMax=[]  FilterDenConstantOutDataTypeStr=Inherit: Inherit via back propagation  FilterDenConstantOutMin=[]  FilterDenConstantOutMax=[]  PCopyOutDataTypeStr=Inherit: Inherit via back propagation  PCopyOutMin=[]  PCopyOutMax=[]  NCopyOutDataTypeStr=Inherit: Inherit via back propagation  NCopyOutMin=[]  NCopyOutMax=[]  IntegratorContinuousStateAttributes=''  IntegratorStateMustResolveToSignalObject=off  IntegratorRTWStateStorageClass=Auto  FilterContinuousStateAttributes=''  FilterStateMustResolveToSignalObject=off  FilterRTWStateStorageClass=Auto  ParallelPVariant=InternalParameters  IdealPVariant=Disabled  IVariant=InternalParameters  DVariant=Disabled  IntegratorVariant=Discrete  SatVariant=Enabled  AWVariant=BackCalculation  PCopyVariant=Disabled  TRVariant=Disabled  FdbkBlocksVariant=Feedback  IdealPFdbkVariant=Passthrough  SatFdbkVariant=Enabled  DerivativeFilterVariant=Disabled  NVariant=Disabled  NCopyVariant=Disabled_SignalSpec  FilterICVariant=Disabled  IntegratorICVariant=InternalICs  ExternalResetVariant=Disabled  TRSumVariant=Passthrough  SumFdbkVariant=Enabled  SumVariant=Sum_PI  TsampFilterVariant=InternalTs  TsampNgainVariant=Passthrough  TsampIntegralVariant=Disabled_SignalSpec  ExternalSaturationOutDataTypeStr=Inherit: Same as second input  DerivativeSourceVariant=Disabled  PreIntVariant=InternalPreInt
  PWM Generation : pwm_cpulib/PWM Generation  f_FPGA=1/ts_FPGA_clk  n_channels=1  sel_scaling=CPU  protection_param=Disabled: A and B can be high at the same moment  deadband_sec=PFC_PWM_Deadband  natural_update=At period starts  delay=0  trigger_duration_sec=[1e-6]  trigger_period_start=off  trigger_half_of_the_period=off  trigger_a_on=off  trigger_a_off=off  trigger_b_on=off  trigger_b_off=off  bit_width_pwm_gen=PFC_PWM_BitWidth  invert_a=off  invert_b=off  invert_c=off  showPhaseInput=off
      settings: SourceProductName=PWM CPU Library
  PWM period1 : Constant  Value=1/totemPole.SwitchingFrequency  SampleTime=ts_CPU
  Product : Product
  Sat_Pwr : Saturate  UpperLimit=PFC_Sat_Pwr_Upper  LowerLimit=PFC_Sat_Pwr_Lower
  Sat_iL : Saturate  UpperLimit=PFC_Sat_iL_Upper  LowerLimit=PFC_Sat_iL_Lower
  Saturation_DC : Saturate  UpperLimit=PFC_Sat_DC_Upper  LowerLimit=PFC_Sat_DC_Lower
  Sum1 : Sum  Inputs=|+-
  Sum7 : Sum  Inputs=|+-
  Sum_DC : Sum
  Sum_FF : Sum  Inputs=+-
  PWM_Config_PFC : Outport  VectorParamsAs1DForOutWhenUnconnected=off
  PWM_Runtime_PFC : Outport  Port=2  VectorParamsAs1DForOutWhenUnconnected=off
  wires:
  Abs/1 -> Gain/1, Divide_FF/1
  Gain/1 -> Product/1
  Sum1/1 -> PI Voltage/1
  Abs1/1 -> Sum7/2
  Measured bus voltage/1 -> Sum1/2, Divide_FF/2
  Source voltage/1 -> Abs/1
  Measured inductor current/1 -> Abs1/1
  Reference bus voltage/1 -> Sum1/1
  Sum7/1 -> PI current/1
  PWM period1/1 -> PWM Generation/1
  PWM Generation/2 -> PWM_Runtime_PFC/1
  OL_Switch/1 -> PWM Generation/2  "DC"
  PWM Generation/1 -> PWM_Config_PFC/1
  One/1 -> Sum_FF/1
  Divide_FF/1 -> Sum_FF/2
  Sum_FF/1 -> Sum_DC/1
  PI Voltage/1 -> Sat_Pwr/1
  Sat_Pwr/1 -> Product/2
  Product/1 -> Sat_iL/1
  Sat_iL/1 -> Sum7/1  "iL_ref1"
  PI current/1 -> Sum_DC/2
  Sum_DC/1 -> Saturation_DC/1
  Saturation_DC/1 -> OL_Switch/3
  OpenLoopDuty/1 -> OL_Switch/1
  OpenLoopEnable/1 -> OL_Switch/2

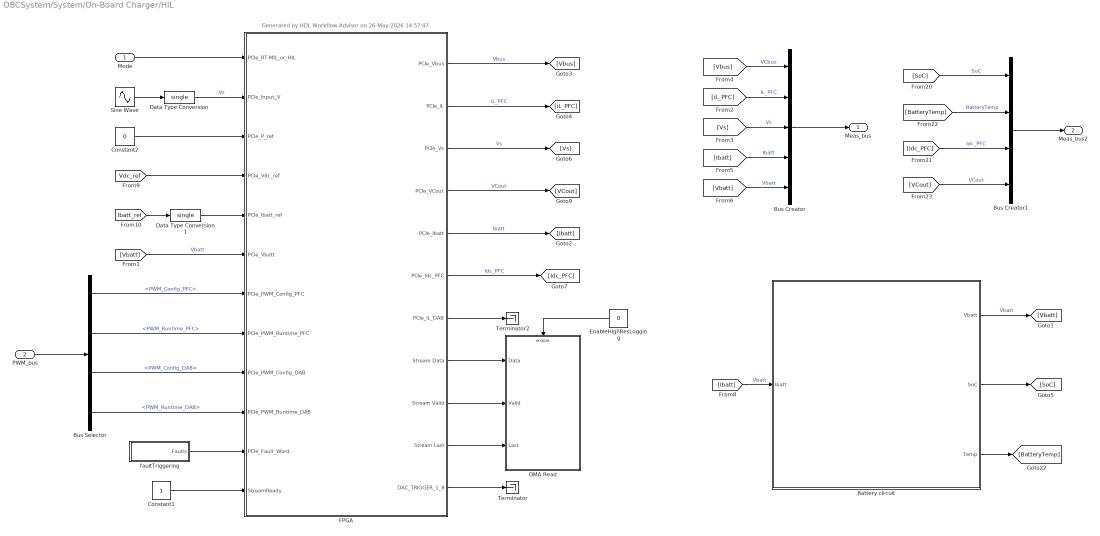
== system OBCSystem/System/On-Board Charger/HIL ==
  note: Generated by HDL Workflow Advisor on 26-May-2026 14:57:47
  Mode : Inport
  PWM_bus : Inport  Port=2
  Battery circuit : Subsystem
      mask Display: image('OnboardChargerBattery.png');
  Bus Creator : BusCreator  Inputs=5
  Bus Creator1 : BusCreator  Inputs=4
  Bus Selector : BusSelector  OutputSignals=PWM_Config_PFC,PWM_Runtime_PFC,PWM_Config_DAB,PWM_Runtime_DAB
  Constant1 : Constant  OutDataTypeStr=boolean  SampleTime=ts_CPU
  Constant2 : Constant  Value=0  OutDataTypeStr=single  SampleTime=ts_CPU
  DMA Read : Subsystem  VariantControl=Real-Time
  Data Type Conversion : DataTypeConversion  OutDataTypeStr=single  SaturateOnIntegerOverflow=off  RndMeth=Floor
  Data Type Conversion1 : DataTypeConversion  OutDataTypeStr=single  SaturateOnIntegerOverflow=off  RndMeth=Floor
  EnableHighResLogging : Constant  Value=0  OutDataTypeStr=boolean  SampleTime=ts_CPU
  FPGA : Subsystem  mask(Speedgoat IO334-325k Interface Block){module_id=1, slot=-1, ts=-1, dacGain_1=+/- 10.0V, dacActiv_1=on, dacInit_1=0, dacGain_2=+/- 10.0V, dacActiv_2=on, dacInit_2=0, dacGain_3=+/- 10.0V, dacActiv_3=on, dacInit_3=0, dacGain_4=+/- 10.0V, dacActiv_4=on, dacInit_4=0, dacGain_5=+/- 10.0V, dacActiv_5=on, dacInit_5=0, dacGain_6=+/- 10.0V, dacActiv_6=on, dacInit_6=0, dacGain_7=+/- 10.0V, dacActiv_7=on, dacInit_7=0, dacGain_8=+/- 10.0V, dacActiv_8=on, dacInit_8=0, dacGain_9=+/- 10.0V, dacActiv_9=off, dacInit_9=0, dacGain_10=+/- 10.0V, dacActiv_10=off, dacInit_10=0, dacGain_11=+/- 10.0V, dacActiv_11=off, dacInit_11=0, dacGain_12=+/- 10.0V, dacActiv_12=off, dacInit_12=0, dacGain_13=+/- 10.0V, dacActiv_13=off, dacInit_13=0, dacGain_14=+/- 10.0V, dacActiv_14=off, dacInit_14=0, dacGain_15=+/- 10.0V, dacActiv_15=off, dacInit_15=0, dacGain_16=+/- 10.0V, dacActiv_16=off, dacInit_16=0, dacGain_17=+/- 10.0V, dacActiv_17=off, dacInit_17=0, dacGain_18=+/- 10.0V, dacActiv_18=off, dacInit_18=0, dacGain_19=+/- 10.0V, dacActiv_19=off, dacInit_19=0, dacGain_20=+/- 10.0V, dacActiv_20=off, dacInit_20=0, dacGain_21=+/- 10.0V, dacActiv_21=off, dacInit_21=0, dacGain_22=+/- 10.0V, dacActiv_22=off, dacInit_22=0, dacGain_23=+/- 10.0V, dacActiv_23=off, dacInit_23=0, dacGain_24=+/- 10.0V, dacActiv_24=off, dacInit_24=0, dacGain_25=+/- 10.0V, dacActiv_25=off, dacInit_25=0, dacGain_26=+/- 10.0V, dacActiv_26=off, dacInit_26=0, dacGain_27=+/- 10.0V, dacActiv_27=off, dacInit_27=0, dacGain_28=+/- 10.0V, dacActiv_28=off, dacInit_28=0, dacGain_29=+/- 10.0V, dacActiv_29=off, dacInit_29=0, dacGain_30=+/- 10.0V, dacActiv_30=off, dacInit_30=0, dacGain_31=+/- 10.0V, dacActiv_31=off, dacInit_31=0, dacGain_32=+/- 10.0V, dacActiv_32=off, dacInit_32=0, dacReset=on, fpga_sync_mode=on, reset_mode=on, reset_mode_stop=on, FpgaFreq=100}
      mask prompts: module_id "FPGA Module Identifier:"; slot "PCI slot (-1: autosearch):"; ts "Sample time:"; dacGain_1 "DAC Ch 01 Range"; dacActiv_1 "Active"; dacInit_1 "Initial Value"; dacGain_2 "DAC Ch 02 Range"; dacActiv_2 "Active"; dacInit_2 "Initial Value"; dacGain_3 "DAC Ch 03 Range"; dacActiv_3 "Active"; dacInit_3 "Initial Value"; dacGain_4 "DAC Ch 04 Range"; dacActiv_4 "Active"; dacInit_4 "Initial Value"; dacGain_5 "DAC Ch 05 Range"; dacActiv_5 "Active"; dacInit_5 "Initial Value"; dacGain_6 "DAC Ch 06 Range"; dacActiv_6 "Active"; dacInit_6 "Initial Value"; dacGain_7 "DAC Ch 07 Range"; dacActiv_7 "Active"; dacInit_7 "Initial Value"; dacGain_8 "DAC Ch 08 Range"; dacActiv_8 "Active"; dacInit_8 "Initial Value"; dacGain_9 "DAC Ch 09 Range"; dacActiv_9 "Active"; dacInit_9 "Initial Value"; dacGain_10 "DAC Ch 10 Range"; dacActiv_10 "Active"; dacInit_10 "Initial Value"; dacGain_11 "DAC Ch 11 Range"; dacActiv_11 "Active"; dacInit_11 "Initial Value"; dacGain_12 "DAC Ch 12 Range"; dacActiv_12 "Active"; dacInit_12 "Initial Value"; dacGain_13 "DAC Ch 13 Range"; dacActiv_13 "Active"; dacInit_13 "Initial Value"; dacGain_14 "DAC Ch 14 Range"; dacActiv_14 "Active"; dacInit_14 "Initial Value"; dacGain_15 "DAC Ch 15 Range"; dacActiv_15 "Active"; dacInit_15 "Initial Value"; dacGain_16 "DAC Ch 16 Range"; dacActiv_16 "Active"; dacInit_16 "Initial Value"; dacGain_17 "DAC Ch 17 Range"; dacActiv_17 "Active"; dacInit_17 "Initial Value"; dacGain_18 "DAC Ch 18 Range"; dacActiv_18 "Active"; dacInit_18 "Initial Value"; dacGain_19 "DAC Ch 19 Range"; dacActiv_19 "Active"; dacInit_19 "Initial Value"; dacGain_20 "DAC Ch 20 Range"; dacActiv_20 "Active"; dacInit_20 "Initial Value"; dacGain_21 "DAC Ch 21 Range"; dacActiv_21 "Active"; dacInit_21 "Initial Value"; dacGain_22 "DAC Ch 22 Range"; dacActiv_22 "Active"; dacInit_22 "Initial Value"; dacGain_23 "DAC Ch 23 Range"; dacActiv_23 "Active"; dacInit_23 "Initial Value"; dacGain_24 "DAC Ch 24 Range"; dacActiv_24 "Active"; dacInit_24 "Initial Value"; dacGain_25 "DAC Ch 25 Range"; dacActiv_25 "Active"; dacInit_25 "Initial Value"; dacGain_26 "DAC Ch 26 Range"; dacActiv_26 "Active"; dacInit_26 "Initial Value"; dacGain_27 "DAC Ch 27 Range"; dacActiv_27 "Active"; dacInit_27 "Initial Value"; dacGain_28 "DAC Ch 28 Range"; dacActiv_28 "Active"; dacInit_28 "Initial Value"; dacGain_29 "DAC Ch 29 Range"; dacActiv_29 "Active"; dacInit_29 "Initial Value"; dacGain_30 "DAC Ch 30 Range"; dacActiv_30 "Active"; dacInit_30 "Initial Value"; dacGain_31 "DAC Ch 31 Range"; dacActiv_31 "Active"; dacInit_31 "Initial Value"; dacGain_32 "DAC Ch 32 Range"; dacActiv_32 "Active"; dacInit_32 "Initial Value"; dacReset "Reset to initial value at model stop"; fpga_sync_mode "Run FPGA only when target application runs"; reset_mode "Reset FPGA states on start"; reset_mode_stop "Reset FPGA states on stop"; FpgaFreq "FPGA Frequency [MHz]"
      mask help: Simulink Real-Time Interface Block for Speedgoat IO334-325k.
      mask init:
      | hdlslrt.backend.mfpgaparameters;
      | if sg.hdlc.utils.compareMatlabVersion('~=', 'R2025b')
      | 	sg.hdlc.warning(['The interface model that you are attempting to use was generated ',...
      | 		'in MATLAB R2025b and may not be compatible with the version you are currently using. ',...
      | 		'Attempting to use this interface model in a different MATLAB release can lead to ',...
      | 		'application crashes or other unpredictable behavior. ',...
      | 		'In order to avoid this and ensure stability and correct functionality, ',...
      | 		'we highly recommend regenerating the model with your current MATLAB release.']);
      | end
      mask Help: eval('sg.hdlc.utils.help.show(''refentry_workflow_generated_model'',''isHdlcHelp'', true)')
      mask TypeOptions dacGain_1: AD5547 Setup/dacGain_1
      mask TypeOptions dacActiv_1: AD5547 Setup/dacActiv_1
      mask TypeOptions dacInit_1: AD5547 Setup/dacInit_1
      mask TypeOptions dacGain_2: AD5547 Setup/dacGain_2
      mask TypeOptions dacActiv_2: AD5547 Setup/dacActiv_2
      mask TypeOptions dacInit_2: AD5547 Setup/dacInit_2
      mask TypeOptions dacGain_3: AD5547 Setup/dacGain_3
      mask TypeOptions dacActiv_3: AD5547 Setup/dacActiv_3
      mask TypeOptions dacInit_3: AD5547 Setup/dacInit_3
      mask TypeOptions dacGain_4: AD5547 Setup/dacGain_4
      mask TypeOptions dacActiv_4: AD5547 Setup/dacActiv_4
      mask TypeOptions dacInit_4: AD5547 Setup/dacInit_4
      mask TypeOptions dacGain_5: AD5547 Setup/dacGain_5
      mask TypeOptions dacActiv_5: AD5547 Setup/dacActiv_5
      mask TypeOptions dacInit_5: AD5547 Setup/dacInit_5
      mask TypeOptions dacGain_6: AD5547 Setup/dacGain_6
      mask TypeOptions dacActiv_6: AD5547 Setup/dacActiv_6
      mask TypeOptions dacInit_6: AD5547 Setup/dacInit_6
      mask TypeOptions dacGain_7: AD5547 Setup/dacGain_7
      mask TypeOptions dacActiv_7: AD5547 Setup/dacActiv_7
      mask TypeOptions dacInit_7: AD5547 Setup/dacInit_7
      mask TypeOptions dacGain_8: AD5547 Setup/dacGain_8
      mask TypeOptions dacActiv_8: AD5547 Setup/dacActiv_8
      mask TypeOptions dacInit_8: AD5547 Setup/dacInit_8
      mask TypeOptions dacGain_9: AD5547 Setup/dacGain_9
      mask TypeOptions dacActiv_9: AD5547 Setup/dacActiv_9
      mask TypeOptions dacInit_9: AD5547 Setup/dacInit_9
      mask TypeOptions dacGain_10: AD5547 Setup/dacGain_10
      mask TypeOptions dacActiv_10: AD5547 Setup/dacActiv_10
      mask TypeOptions dacInit_10: AD5547 Setup/dacInit_10
      mask TypeOptions dacGain_11: AD5547 Setup/dacGain_11
      mask TypeOptions dacActiv_11: AD5547 Setup/dacActiv_11
      mask TypeOptions dacInit_11: AD5547 Setup/dacInit_11
      mask TypeOptions dacGain_12: AD5547 Setup/dacGain_12
      mask TypeOptions dacActiv_12: AD5547 Setup/dacActiv_12
      mask TypeOptions dacInit_12: AD5547 Setup/dacInit_12
      mask TypeOptions dacGain_13: AD5547 Setup/dacGain_13
      mask TypeOptions dacActiv_13: AD5547 Setup/dacActiv_13
      mask TypeOptions dacInit_13: AD5547 Setup/dacInit_13
      mask TypeOptions dacGain_14: AD5547 Setup/dacGain_14
      mask TypeOptions dacActiv_14: AD5547 Setup/dacActiv_14
      mask TypeOptions dacInit_14: AD5547 Setup/dacInit_14
      mask TypeOptions dacGain_15: AD5547 Setup/dacGain_15
      mask TypeOptions dacActiv_15: AD5547 Setup/dacActiv_15
      mask TypeOptions dacInit_15: AD5547 Setup/dacInit_15
      mask TypeOptions dacGain_16: AD5547 Setup/dacGain_16
      mask TypeOptions dacActiv_16: AD5547 Setup/dacActiv_16
      mask TypeOptions dacInit_16: AD5547 Setup/dacInit_16
      mask TypeOptions dacGain_17: AD5547 Setup/dacGain_17
      mask TypeOptions dacActiv_17: AD5547 Setup/dacActiv_17
      mask TypeOptions dacInit_17: AD5547 Setup/dacInit_17
      mask TypeOptions dacGain_18: AD5547 Setup/dacGain_18
      mask TypeOptions dacActiv_18: AD5547 Setup/dacActiv_18
      mask TypeOptions dacInit_18: AD5547 Setup/dacInit_18
      mask TypeOptions dacGain_19: AD5547 Setup/dacGain_19
      mask TypeOptions dacActiv_19: AD5547 Setup/dacActiv_19
      mask TypeOptions dacInit_19: AD5547 Setup/dacInit_19
      mask TypeOptions dacGain_20: AD5547 Setup/dacGain_20
      mask TypeOptions dacActiv_20: AD5547 Setup/dacActiv_20
      mask TypeOptions dacInit_20: AD5547 Setup/dacInit_20
      mask TypeOptions dacGain_21: AD5547 Setup/dacGain_21
      mask TypeOptions dacActiv_21: AD5547 Setup/dacActiv_21
      mask TypeOptions dacInit_21: AD5547 Setup/dacInit_21
      mask TypeOptions dacGain_22: AD5547 Setup/dacGain_22
      mask TypeOptions dacActiv_22: AD5547 Setup/dacActiv_22
      mask TypeOptions dacInit_22: AD5547 Setup/dacInit_22
      mask TypeOptions dacGain_23: AD5547 Setup/dacGain_23
      mask TypeOptions dacActiv_23: AD5547 Setup/dacActiv_23
      mask TypeOptions dacInit_23: AD5547 Setup/dacInit_23
      mask TypeOptions dacGain_24: AD5547 Setup/dacGain_24
      mask TypeOptions dacActiv_24: AD5547 Setup/dacActiv_24
      mask TypeOptions dacInit_24: AD5547 Setup/dacInit_24
      mask TypeOptions dacGain_25: AD5547 Setup/dacGain_25
      mask TypeOptions dacActiv_25: AD5547 Setup/dacActiv_25
      mask TypeOptions dacInit_25: AD5547 Setup/dacInit_25
      mask TypeOptions dacGain_26: AD5547 Setup/dacGain_26
      mask TypeOptions dacActiv_26: AD5547 Setup/dacActiv_26
      mask TypeOptions dacInit_26: AD5547 Setup/dacInit_26
      mask TypeOptions dacGain_27: AD5547 Setup/dacGain_27
      mask TypeOptions dacActiv_27: AD5547 Setup/dacActiv_27
      mask TypeOptions dacInit_27: AD5547 Setup/dacInit_27
      mask TypeOptions dacGain_28: AD5547 Setup/dacGain_28
      mask TypeOptions dacActiv_28: AD5547 Setup/dacActiv_28
      mask TypeOptions dacInit_28: AD5547 Setup/dacInit_28
      mask TypeOptions dacGain_29: AD5547 Setup/dacGain_29
      mask TypeOptions dacActiv_29: AD5547 Setup/dacActiv_29
      mask TypeOptions dacInit_29: AD5547 Setup/dacInit_29
      mask TypeOptions dacGain_30: AD5547 Setup/dacGain_30
      mask TypeOptions dacActiv_30: AD5547 Setup/dacActiv_30
      mask TypeOptions dacInit_30: AD5547 Setup/dacInit_30
      mask TypeOptions dacGain_31: AD5547 Setup/dacGain_31
      mask TypeOptions dacActiv_31: AD5547 Setup/dacActiv_31
      mask TypeOptions dacInit_31: AD5547 Setup/dacInit_31
      mask TypeOptions dacGain_32: AD5547 Setup/dacGain_32
      mask TypeOptions dacActiv_32: AD5547 Setup/dacActiv_32
      mask TypeOptions dacInit_32: AD5547 Setup/dacInit_32
      mask TypeOptions dacReset: AD5547 Setup/dacReset
      mask TypeOptions fpga_sync_mode: IO3xx Setup/fpga_sync_mode
      mask TypeOptions reset_mode: IO3xx Setup/reset_mode
      mask TypeOptions reset_mode_stop: IO3xx Setup/reset_mode_stop
      mask DialogControl DAC Prompt: DAC
      mask DialogControl dacGrp_1 Prompt: Ch 01 to 08
      mask DialogControl dacGrp_2 Prompt: Ch 09 to 16
      mask DialogControl dacGrp_3 Prompt: Ch 17 to 24
      mask DialogControl dacGrp_4 Prompt: Ch 25 to 32
      mask Display:
      | SetupBlkPath = sghdlc.model.findSystem(gcb, 'LookUnderMasks', 'all', 'FollowLinks', 'on', 'regexp', 'on', 'Name', 'IO3(\d|x){2}\s+Setup' );
      | SetupBlkPath = SetupBlkPath{1};
      | TS = get_param(SetupBlkPath,'timestamp_mcs');
      | disp(sprintf('Speedgoat IO334-325k\n\nTimestamp\n%s\n\nReference Design\nVersion 1.1\n\nMATLAB R2025b\n\nPCIe Link Width: X4\nTiming Severity: error\nRear Plugin: None\nAurora Mode: None\nAurora Crc: true\nAurora Byteswap: true\nVerifier: off\nVerifier: JTAG\n', TS))
  Sine Wave : Sin  Amplitude=grid.ACVoltageRMS*sqrt(2)  Frequency=grid.SystemFrequency*2*pi  Phase=-ts_CPU/grid.SystemFrequency*2*pi*0  SampleTime=ts_CPU
  Terminator : Terminator
  Terminator2 : Terminator
  faultTriggering : Subsystem
  Meas_bus : Outport
  Meas_bus2 : Outport  Port=2
  wires:
  Mode/1 -> FPGA/1(PCIe_RT-MIL_or_HIL)
  FPGA/1(PCIe_Vbus) -> [Vbus]  "Vbus"
  FPGA/2(PCIe_iL) -> [iL_PFC]  "iL_PFC"
  FPGA/3(PCIe_Vs) -> [Vs]  "Vs"
  [Vdc_ref] -> FPGA/4(PCIe_Vdc_ref)
  [Vbatt] -> FPGA/6(PCIe_Vbatt)  "Vbatt"
  FPGA/4(PCIe_VCout) -> [VCout]  "VCout"
  FPGA/6(PCIe_Idc_PFC) -> [Idc_PFC]  "Idc_PFC"
  faultTriggering/1(Faults) -> FPGA/11(PCIe_Fault_Word)
  FPGA/10(Stream Last) -> DMA Read/3(Last)
  FPGA/5(PCIe_Ibatt) -> [Ibatt]  "Ibatt"
  Sine Wave/1 -> Data Type Conversion/1
  Data Type Conversion/1 -> FPGA/2(PCIe_Input_V)  "Vs"
  EnableHighResLogging/1 -> DMA Read/Enable
  Bus Creator/1 -> Meas_bus/1
  [Vbus] -> Bus Creator/1  "VCbus"
  [iL_PFC] -> Bus Creator/2  "iL_PFC"
  [Vs] -> Bus Creator/3  "Vs"
  [Ibatt] -> Bus Creator/4  "Ibatt"
  [Vbatt] -> Bus Creator/5  "Vbatt"
  Battery circuit/1(Vbatt) -> [Vbatt]  "Vbatt"
  [Ibatt] -> Battery circuit/1(Ibatt)  "Vbatt"
  PWM_bus/1 -> Bus Selector/1
  Bus Selector/1 -> FPGA/7(PCIe_PWM_Config_PFC)  "<PWM_Config_PFC>"
  Bus Selector/2 -> FPGA/8(PCIe_PWM_Runtime_PFC)  "<PWM_Runtime_PFC>"
  Bus Selector/3 -> FPGA/9(PCIe_PWM_Config_DAB)  "<PWM_Config_DAB>"
  Bus Selector/4 -> FPGA/10(PCIe_PWM_Runtime_DAB)  "<PWM_Runtime_DAB>"
  [Ibatt_ref] -> Data Type Conversion1/1
  [BatteryTemp] -> Bus Creator1/2  "BatteryTemp"
  [VCout] -> Bus Creator1/4  "VCout"
  [Idc_PFC] -> Bus Creator1/3  "Idc_PFC"
  Bus Creator1/1 -> Meas_bus2/1
  [SoC] -> Bus Creator1/1  "SoC"
  Battery circuit/2(SoC) -> [SoC]
  Battery circuit/3(Temp) -> [BatteryTemp]
  FPGA/9(Stream Valid) -> DMA Read/2(Valid)
  Constant1/1 -> FPGA/12(StreamReady)
  FPGA/8(Stream Data) -> DMA Read/1(Data)
  FPGA/11(DAC_TRIGGER_1_8) -> Terminator/1
  Data Type Conversion1/1 -> FPGA/5(PCIe_Ibatt_ref)
  Constant2/1 -> FPGA/3(PCIe_P_ref)
  FPGA/7(PCIe_iL_DAB) -> Terminator2/1

== system OBCSystem/System/On-Board Charger/MIL ==
  PWM_bus : Inport
  Bus Selector : BusSelector  OutputSignals=PWM_Config_PFC,PWM_Runtime_PFC,PWM_Config_DAB,PWM_Runtime_DAB
  PWM : Subsystem
  Rate Transition3 : RateTransition  OutPortSampleTime=ts_FPGA_mdl
  Simscape : Subsystem  VariantControl=strcmp(get_param(getfullname(Simulink.findBlocks(bdroot,'Name','SimulationMode')),'value'),'0')
      mask Display: image('OnboardChargerSchematics.png');
  Meas_bus : Outport
  Meas_bus2 : Outport  Port=2
  wires:
  Simscape/1(Out1) -> Meas_bus/1
  PWM/1(Out1) -> Simscape/1(Gates)
  PWM_bus/1 -> Rate Transition3/1
  Bus Selector/1 -> PWM/1(PWM_Config)  "<PWM_Config_PFC>"
  Bus Selector/2 -> PWM/2(PWM_Runtime)  "<PWM_Runtime_PFC>"
  Bus Selector/3 -> PWM/3(Configuration)  "<PWM_Config_DAB>"
  Bus Selector/4 -> PWM/4(Runtime_CPU)  "<PWM_Runtime_DAB>"
  Rate Transition3/1 -> Bus Selector/1
  Simscape/2(Out2) -> Meas_bus2/1

== system OBCSystem/User Interface/Instrumentation/Fourier ==
  In : Inport
  Fourier Analysis : eeGeneralControl/Fourier Analysis  f=50  n=0  M0=Fourier_class([0 0]).objParamMappingDerived.NewDerivedParam.M0  Ph0=Fourier_class([0 0]).objParamMappingDerived.NewDerivedParam.Ph0  BufferSize=8192  Ts=ts_CPU
  Gain : Gain  Gain=180/pi
  Mag : Outport  VectorParamsAs1DForOutWhenUnconnected=off
  Phase : Outport  Port=2  VectorParamsAs1DForOutWhenUnconnected=off
  wires:
  Gain/1 -> Phase/1
  Fourier Analysis/2 -> Gain/1
  Fourier Analysis/1 -> Mag/1
  In/1 -> Fourier Analysis/1
